simulink model "Test_Linearisation"  (R2024b)
settings: Solver=VariableStepAuto  StartTime=0.0  StopTime=20  RelTol=1e-3
settings Model: Creator=GH-X-ST  LastModifiedBy=GH-X-ST

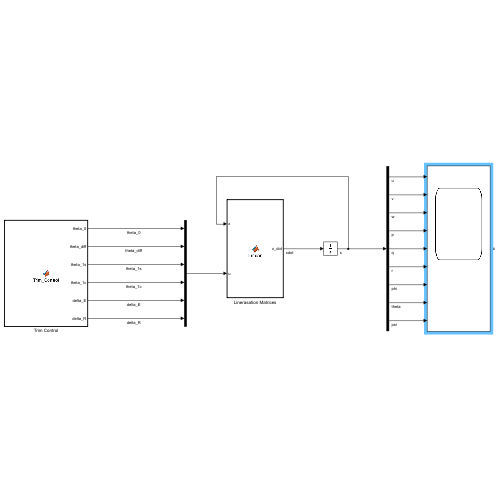
[thumbnail: Simulink's stored preview of the top-level diagram]
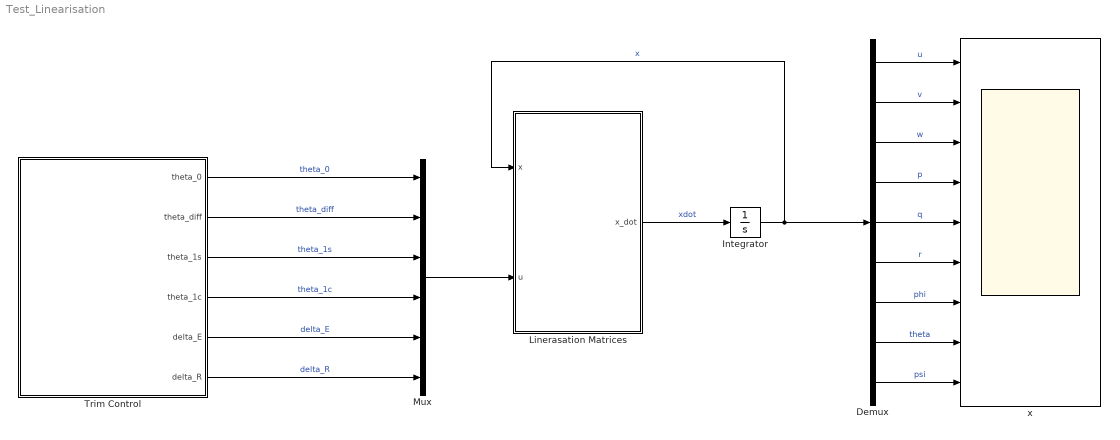
== system Test_Linearisation ==
  Demux : Demux  Outputs=9
  Integrator : Integrator  InitialCondition=[0;0;0;0;0;0;0;0;0]
  Linerasation Matrices : MATLAB Function  TreatAsAtomicUnit=on
  Mux : Mux  Inputs=6
  Trim Control : MATLAB Function  TreatAsAtomicUnit=on
  x : Scope  NumInputPorts=9
  wires:
  Mux/1 -> Linerasation Matrices/2(u)
  Trim Control/1(theta_0) -> Mux/1  "theta_0"
  Trim Control/2(theta_diff) -> Mux/2  "theta_diff"
  Trim Control/3(theta_1s) -> Mux/3  "theta_1s"
  Trim Control/4(theta_1c) -> Mux/4  "theta_1c"
  Trim Control/5(delta_E) -> Mux/5  "delta_E"
  Trim Control/6(delta_R) -> Mux/6  "delta_R"
  Integrator/1 -> Demux/1, Linerasation Matrices/1(x)  "x"
  Linerasation Matrices/1(x_dot) -> Integrator/1  "xdot"
  Demux/1 -> x/1  "u"
  Demux/2 -> x/2  "v"
  Demux/3 -> x/3  "w"
  Demux/4 -> x/4  "p"
  Demux/5 -> x/5  "q"
  Demux/6 -> x/6  "r"
  Demux/7 -> x/7  "phi"
  Demux/8 -> x/8  "theta"
  Demux/9 -> x/9  "psi"

== matlab function Test_Linearisation/Trim Control ==
  data: theta_0 output; theta_diff output; theta_1s output; theta_1c output; delta_E output; delta_R output
function [theta_0, theta_diff, theta_1s, theta_1c, delta_E, delta_R] = Trim_Control
% Author:
%   Hanchen Li (hl3422@ic.ac.uk)

% ctrl_trans = [0.166120634642684	-0.00650795728853242	-0.0578853588811545	-0.0189229713146117	-0.00711805187731994	0.000379045090706055];

ctrl_trans = [0, 0, 0, 0, 0, 0];

theta_0 = ctrl_trans(1);

theta_diff = ctrl_trans(2);

theta_1s = ctrl_trans(3);

theta_1c = ctrl_trans(4);

delta_E = ctrl_trans(5);

delta_R = ctrl_trans(6);

end

== matlab function Test_Linearisation/Linerasation Matrices ==
  data: x input; u input; x_dot output
function x_dot = Linear(x, u)
% Author:
%   Hanchen Li (hl3422@ic.ac.uk)

A = ...
[0.00198907487199834	0.00253061362903012	0.00124807180451603	-0.692167063514638	-1.31545814391634	0	0	-9.77936080280246	0;
-0.00588447670188397	-0.113487618299962	0.0638672384599415	-0.474169631164562	0.334103423678539	-72.0222222000000	9.80530163216295	-0.000810364497449978	0;
0.208959151679622	-0.0211851542974983	-2.91377790533787	0.774705894759364	74.4525040940847	0	-0.154237243847888	-0.690902155824347	0;
-0.184449747074291	0.186394218922800	7.40087985212333	-44.6707815075849	-71.0404373967689	0	0	0	0;
-0.00261903529268842	-0.0419495664042437	0.0663122914709030	3.04300170848933	-1.76288467057787	0	0	0	0;
-0.0708839132123084	0.0441186726466513	2.83701124102899	-17.1062286441804	-27.1919799107843	0	0	0	0;
0	0	0	1	8.26353223144712e-05	0.00525336319929938	0	0	0;
0	0	0	0	0.999876306745786	-0.0157280389243905	0	0	0;
0	0	0	0	0.0157282560064247	0.999890107270042	0	0	0];

B = ...
[-9.36734534820370	20.1055736208756	-11.2809889940346	8.49863312752986	0	-0.00286205661743227;
7.36311189397626	8.61969410886620	5.51170758593719	3.36925382550327	0	-7.87065569844800;
-257.948569477389	-0.838567623020481	-112.985439522211	-16.5654464419962	-8.64803218389554	0;
515.073062586662	-19.7749208552367	564.154986342246	470.879026333778	0	-6.25148705800775;
-16.7725921688728	-3.05666119991683	-22.1441400308729	17.1904558374243	-3.62798452869815	0.000138246000234776;
197.574622837323	-7.60984268371909	216.152977334537	180.231587049336	0	-4.35740593383498;
0	0	0	0	0	0;
0	0	0	0	0	0;
0	0	0	0	0	0];

%% 3 Output
x_dot = A * x + B * u;

end
